simulink model "motorl"  (R2014b)
settings: Solver=ode23tb  StartTime=0.0  StopTime=1  MaxStep=.0001  MinStep=0.00001  RelTol=1e-3
libraries: powerlib x58, simulink x30, powerlib_extras x2
settings Model: Creator=Muruganandham  LastModifiedBy=SELVA
settings DataIOCC: SignalLoggingSaveFormat=ModelDataLogs
settings OptimizationCC: ExpressionDepthLimit=2147483647
settings DebuggingCC: UnderspecifiedInitializationDetection=Classic  MergeDetectMultiDrivingBlocksExec=none  FcnCallInpInsideContextMsg=UseLocalSettings  StateNameClashWarn=warning
settings GRTTargetCC: CombineOutputUpdateFcns=off  GRTInterface=on

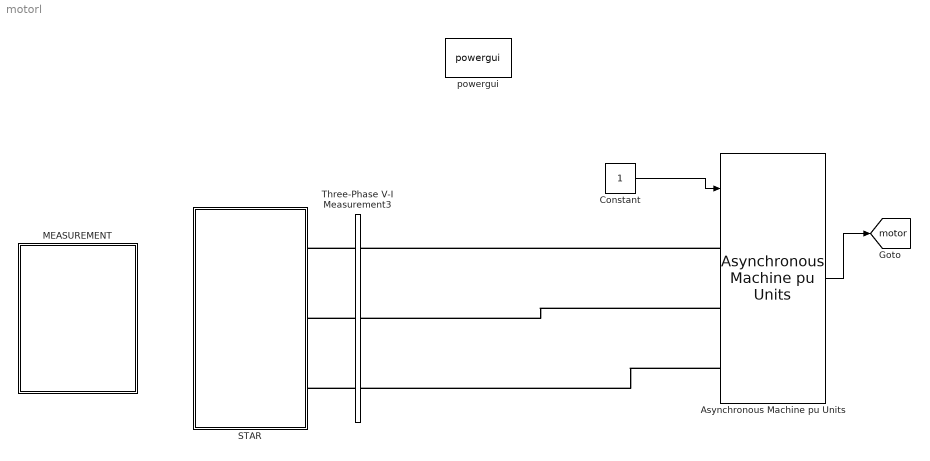
== system motorl ==
  Asynchronous Machine pu Units : powerlib/Machines/Asynchronous Machine pu Units  PresetModel="15:  5.4 HP (4KW)   400 V  50Hz 1430 RPM"  MechanicalLoad=Torque Tm  ShowDetailedParameters=on  RotorType=Squirrel-cage  ReferenceFrame=Rotor  Units=pu  MeasurementBus=off  NominalParameters=[4000 400 50]  Stator=[0.03513 0.04586]  Rotor=[0.03488 0.04586]  Cage1=[0.01909 0.0397]  Cage2=[0.01909 0.0397]  Lm=1.352  Mechanical=[0.0404 0.01841 2]  PolePairs=2  InitialConditions="[ 1,0   0,0,0   0,0,0 ]"  SimulateSaturation=off  Saturation="[0.212,0.4201,0.8125,1.0979,1.4799,2.2457,3.2586,4.5763,6.4763 ;   0.5,0.7,0.9,1,1.1,1.2 ,1.3,1.4,1.5]"  LoadFlowParameters=0  TsPowergui=0  TsBlock=-1  IterativeModel=Trapezoidal non iterative  Pmec=0
  Constant : Constant
  MEASUREMENT : Subsystem
  STAR : Subsystem  mask{v=65, fc=3000, m=1, d=0.0067}
      mask prompts: v "VOLTAGE"; fc "Switching Frequency"; m "Modulation Index"; d "Delay"
  Three-Phase V-I Measurement3 : powerlib/Measurements/Three-Phase V-I Measurement  VoltageMeasurement=phase-to-phase  SetLabelV=on  LabelV=Vabc  Vpu=off  VpuLL=off  CurrentMeasurement=yes  SetLabelI=on  LabelI=Iabc  Ipu=off  Pbase=100e6  Vbase=500e3  OutputType=Complex  PhasorSimulation=off  PSBequivalent=0
  powergui : powerlib/powergui  Priority=1  SimulationMode=Discrete  SolverType=Tustin  SampleTime=50e-6  frequency=60  SPID=off  DisableSnubberDevices=off  DisableRonSwitches=off  DisableVfSwitches=off  SwTol=0  DisplayEquations=off  Interpol=off  methode=off  Ts=0  frequencyindice=0  Pbase=100e6  ErrMax=1e-4  Iterations=50  UnitsV=kV  UnitsW=MW  FunctionMessages=off  echomessages=off  HookPort=off  EnableUseOfTLC=off  x0status=blocks  RestoreLinks=warning  ResistiveCurrentMeasurement=off  Frange=[0:2:500]  Ylog=off  Xlog=on  ShowGrid=off  save=off  variable=ZData  structure=hn  ZoomFFT=off  StartTime=0.04  cycles=7  DisplayStyle=1  fundamental=50  FreqAxis=off  MaxFrequency=1000  frequencyindicesteady=1  RmsSteady=1  display=off
  tag scope: motor=global
  wires:
  Constant/1 -> Asynchronous Machine pu Units/1
  Asynchronous Machine pu Units/1 -> [motor]
  connections:
  Asynchronous Machine pu Units/LConn3 -- Three-Phase V-I Measurement3/LConn3
  Three-Phase V-I Measurement3/RConn3 -- STAR/RConn3
  Asynchronous Machine pu Units/LConn1 -- Three-Phase V-I Measurement3/LConn1
  Three-Phase V-I Measurement3/RConn2 -- STAR/RConn2
  Three-Phase V-I Measurement3/RConn1 -- STAR/RConn1
  Asynchronous Machine pu Units/LConn2 -- Three-Phase V-I Measurement3/LConn2

== system motorl/MEASUREMENT ==
  Bus Selector : BusSelector  OutputSignals=Mechanical.Rotor speed (wm)
  Display1 : Display
  Display3 : Display
  RMS1 : powerlib_extras/Measurements/RMS  f1=50
  RMS2 : powerlib_extras/Measurements/RMS  f1=50
  Scope : Scope
      settings: YMin=-1.16  YMax=-0.96  SaveName=ScopeData5
  Scope1 : Scope
      settings: TimeRange=0.5  YMin=-800  YMax=800  SaveName=bn
  Scope2 : Scope
      settings: TimeRange=0.5  YMin=-30  YMax=30  SaveName=bn1
  wires:
  RMS2/1 -> Display3/1
  [Vabc] -> RMS2/1, Scope1/1
  [motor] -> Bus Selector/1
  Bus Selector/1 -> Scope/1  "<Rotor speed (wm)>"
  RMS1/1 -> Display1/1
  [Iabc] -> RMS1/1, Scope2/1

== system motorl/STAR ==
  "B " : Subsystem
  DC : Subsystem
  DC1 : Subsystem
  DC2 : Subsystem
  Ground : powerlib/Elements/Ground  LConnTagsString=a
  PULSE : Subsystem
  R : Subsystem
  Y : Subsystem
  A : PMIOPort  Tag=PMCPort  Port=1  Side=Right
  B : PMIOPort  Tag=PMCPort  Port=2  Side=Right
  C : PMIOPort  Tag=PMCPort  Port=3  Side=Right
  connections:
  Y/RConn2 -- Ground/LConn1 -- "B "/RConn2 -- R/RConn2
  DC/RConn1 -- R/LConn1
  DC/RConn3 -- R/LConn3
  DC/RConn4 -- R/LConn4
  DC/RConn9 -- R/LConn9
  DC/RConn2 -- R/LConn2
  DC/RConn5 -- R/LConn5
  DC/RConn7 -- R/LConn7
  DC/RConn6 -- R/LConn6
  DC/RConn8 -- R/LConn8
  DC/RConn10 -- R/LConn10
  DC1/RConn1 -- Y/LConn1
  DC1/RConn2 -- Y/LConn2
  DC1/RConn3 -- Y/LConn3
  DC1/RConn4 -- Y/LConn4
  DC1/RConn5 -- Y/LConn5
  DC1/RConn6 -- Y/LConn6
  DC1/RConn7 -- Y/LConn7
  DC1/RConn8 -- Y/LConn8
  DC1/RConn9 -- Y/LConn9
  DC1/RConn10 -- Y/LConn10
  DC2/RConn1 -- "B "/LConn1
  DC2/RConn2 -- "B "/LConn2
  DC2/RConn3 -- "B "/LConn3
  DC2/RConn4 -- "B "/LConn4
  DC2/RConn5 -- "B "/LConn5
  DC2/RConn6 -- "B "/LConn6
  DC2/RConn7 -- "B "/LConn7
  DC2/RConn8 -- "B "/LConn8
  DC2/RConn9 -- "B "/LConn9
  DC2/RConn10 -- "B "/LConn10
  A/RConn1 -- R/RConn1
  B/RConn1 -- Y/RConn1
  C/RConn1 -- "B "/RConn1

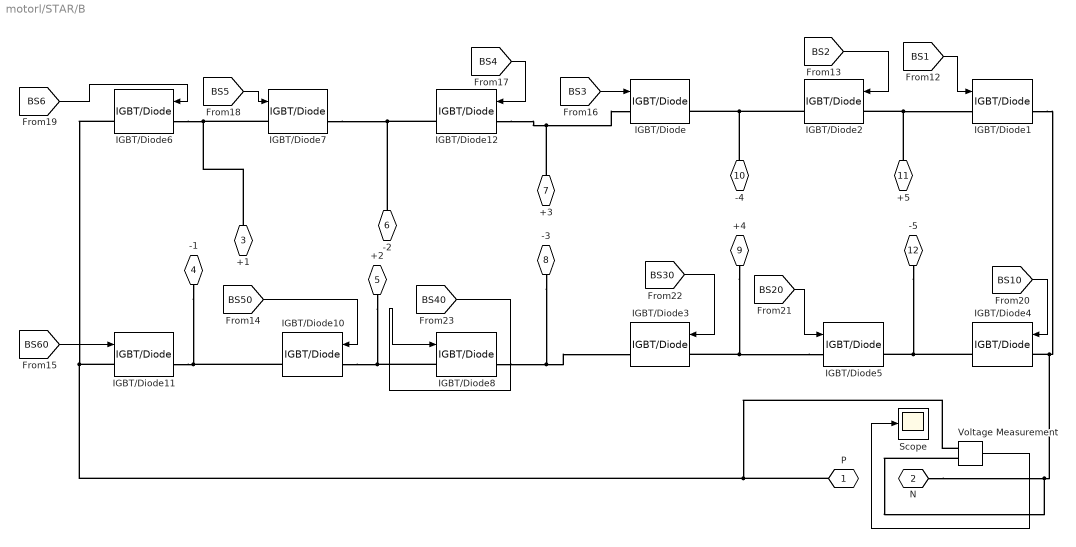
== system motorl/STAR/B  ==
  IGBT/Diode{,1..8,10..12} (12 alike) : powerlib/Power Electronics/IGBT//Diode  Ron=1e-3  Rs=1e5  Cs=inf  Measurements=on
  Scope : Scope
  Voltage Measurement : powerlib/Measurements/Voltage Measurement  PhasorSimulation=off  OutputType=Complex  PSBequivalent=0
  P : PMIOPort  Tag=PMCPort  Port=1  Side=Right
  N : PMIOPort  Tag=PMCPort  Port=2  Side=Right
  +1 : PMIOPort  Tag=PMCPort  Port=3  Side=Left
  -1 : PMIOPort  Tag=PMCPort  Port=4  Side=Left
  +2 : PMIOPort  Tag=PMCPort  Port=5  Side=Left
  -2 : PMIOPort  Tag=PMCPort  Port=6  Side=Left
  +3 : PMIOPort  Tag=PMCPort  Port=7  Side=Left
  -3 : PMIOPort  Tag=PMCPort  Port=8  Side=Left
  +4 : PMIOPort  Tag=PMCPort  Port=9  Side=Left
  -4 : PMIOPort  Tag=PMCPort  Port=10  Side=Left
  +5 : PMIOPort  Tag=PMCPort  Port=11  Side=Left
  -5 : PMIOPort  Tag=PMCPort  Port=12  Side=Left
  wires:
  [BS10] -> IGBT/Diode4/1
  [BS2] -> IGBT/Diode2/1
  [BS20] -> IGBT/Diode5/1
  [BS3] -> IGBT/Diode/1
  [BS30] -> IGBT/Diode3/1
  [BS40] -> IGBT/Diode8/1
  [BS6] -> IGBT/Diode6/1
  [BS4] -> IGBT/Diode12/1
  [BS5] -> IGBT/Diode7/1
  [BS50] -> IGBT/Diode10/1
  [BS60] -> IGBT/Diode11/1
  Voltage Measurement/1 -> Scope/1
  [BS1] -> IGBT/Diode1/1
  connections:
  IGBT/Diode2/RConn1 -- -4/RConn1 -- IGBT/Diode/RConn1
  IGBT/Diode2/LConn1 -- IGBT/Diode1/LConn1 -- +5/RConn1
  IGBT/Diode5/LConn1 -- +4/RConn1 -- IGBT/Diode3/LConn1
  IGBT/Diode4/RConn1 -- -5/RConn1 -- IGBT/Diode5/RConn1
  IGBT/Diode4/LConn1 -- IGBT/Diode1/RConn1 -- N/RConn1 -- Voltage Measurement/LConn2
  IGBT/Diode7/LConn1 -- +1/RConn1 -- IGBT/Diode6/LConn1
  IGBT/Diode12/RConn1 -- IGBT/Diode7/RConn1 -- -2/RConn1
  IGBT/Diode10/RConn1 -- IGBT/Diode11/RConn1 -- -1/RConn1
  IGBT/Diode8/LConn1 -- IGBT/Diode10/LConn1 -- +2/RConn1
  IGBT/Diode12/LConn1 -- IGBT/Diode/LConn1 -- +3/RConn1
  IGBT/Diode8/RConn1 -- IGBT/Diode3/RConn1 -- -3/RConn1
  IGBT/Diode6/RConn1 -- IGBT/Diode11/LConn1 -- P/RConn1 -- Voltage Measurement/LConn1

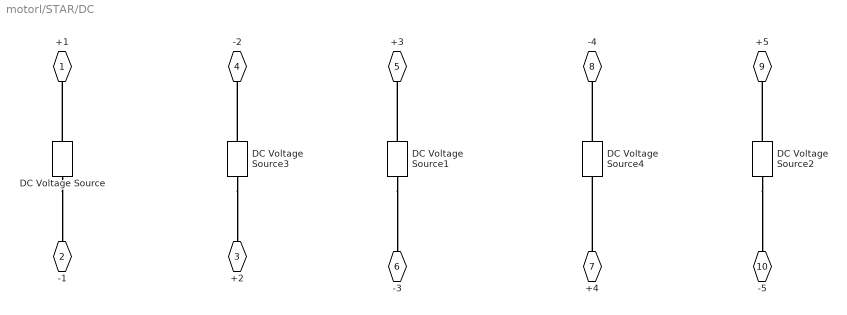
== system motorl/STAR/DC ==
  DC Voltage Source{,1..4} (5 alike) : powerlib/Electrical Sources/DC Voltage Source  Amplitude=v  Measurements=None
  +1 : PMIOPort  Tag=PMCPort  Port=1  Side=Right
  -1 : PMIOPort  Tag=PMCPort  Port=2  Side=Right
  +2 : PMIOPort  Tag=PMCPort  Port=3  Side=Right
  -2 : PMIOPort  Tag=PMCPort  Port=4  Side=Right
  +3 : PMIOPort  Tag=PMCPort  Port=5  Side=Right
  -3 : PMIOPort  Tag=PMCPort  Port=6  Side=Right
  +4 : PMIOPort  Tag=PMCPort  Port=7  Side=Right
  -4 : PMIOPort  Tag=PMCPort  Port=8  Side=Right
  +5 : PMIOPort  Tag=PMCPort  Port=9  Side=Right
  -5 : PMIOPort  Tag=PMCPort  Port=10  Side=Right
  connections:
  DC Voltage Source/LConn1 -- -1/RConn1
  DC Voltage Source/RConn1 -- +1/RConn1
  DC Voltage Source1/LConn1 -- -3/RConn1
  +4/RConn1 -- DC Voltage Source4/RConn1
  DC Voltage Source2/LConn1 -- -5/RConn1
  DC Voltage Source1/RConn1 -- +3/RConn1
  DC Voltage Source2/RConn1 -- +5/RConn1
  DC Voltage Source4/LConn1 -- -4/RConn1
  DC Voltage Source3/LConn1 -- -2/RConn1
  DC Voltage Source3/RConn1 -- +2/RConn1

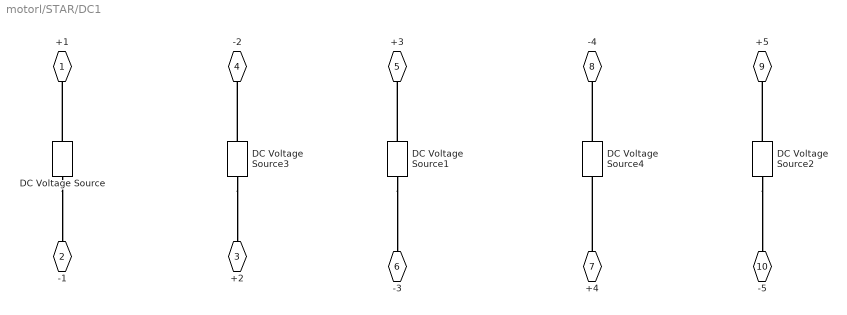
== system motorl/STAR/DC1 ==
  DC Voltage Source{,1..4} (5 alike) : powerlib/Electrical Sources/DC Voltage Source  Amplitude=v  Measurements=None
  +1 : PMIOPort  Tag=PMCPort  Port=1  Side=Right
  -1 : PMIOPort  Tag=PMCPort  Port=2  Side=Right
  +2 : PMIOPort  Tag=PMCPort  Port=3  Side=Right
  -2 : PMIOPort  Tag=PMCPort  Port=4  Side=Right
  +3 : PMIOPort  Tag=PMCPort  Port=5  Side=Right
  -3 : PMIOPort  Tag=PMCPort  Port=6  Side=Right
  +4 : PMIOPort  Tag=PMCPort  Port=7  Side=Right
  -4 : PMIOPort  Tag=PMCPort  Port=8  Side=Right
  +5 : PMIOPort  Tag=PMCPort  Port=9  Side=Right
  -5 : PMIOPort  Tag=PMCPort  Port=10  Side=Right
  connections:
  DC Voltage Source3/RConn1 -- +2/RConn1
  DC Voltage Source3/LConn1 -- -2/RConn1
  DC Voltage Source4/LConn1 -- -4/RConn1
  DC Voltage Source2/RConn1 -- +5/RConn1
  DC Voltage Source1/RConn1 -- +3/RConn1
  DC Voltage Source2/LConn1 -- -5/RConn1
  +4/RConn1 -- DC Voltage Source4/RConn1
  DC Voltage Source1/LConn1 -- -3/RConn1
  DC Voltage Source/RConn1 -- +1/RConn1
  DC Voltage Source/LConn1 -- -1/RConn1

== system motorl/STAR/DC2 ==
  DC Voltage Source{,1..4} (5 alike) : powerlib/Electrical Sources/DC Voltage Source  Amplitude=v  Measurements=None
  +1 : PMIOPort  Tag=PMCPort  Port=1  Side=Right
  -1 : PMIOPort  Tag=PMCPort  Port=2  Side=Right
  +2 : PMIOPort  Tag=PMCPort  Port=3  Side=Right
  -2 : PMIOPort  Tag=PMCPort  Port=4  Side=Right
  +3 : PMIOPort  Tag=PMCPort  Port=5  Side=Right
  -3 : PMIOPort  Tag=PMCPort  Port=6  Side=Right
  +4 : PMIOPort  Tag=PMCPort  Port=7  Side=Right
  -4 : PMIOPort  Tag=PMCPort  Port=8  Side=Right
  +5 : PMIOPort  Tag=PMCPort  Port=9  Side=Right
  -5 : PMIOPort  Tag=PMCPort  Port=10  Side=Right
  connections:
  DC Voltage Source/LConn1 -- -1/RConn1
  DC Voltage Source/RConn1 -- +1/RConn1
  DC Voltage Source1/LConn1 -- -3/RConn1
  +4/RConn1 -- DC Voltage Source4/RConn1
  DC Voltage Source2/LConn1 -- -5/RConn1
  DC Voltage Source1/RConn1 -- +3/RConn1
  DC Voltage Source2/RConn1 -- +5/RConn1
  DC Voltage Source4/LConn1 -- -4/RConn1
  DC Voltage Source3/LConn1 -- -2/RConn1
  DC Voltage Source3/RConn1 -- +2/RConn1

== system motorl/STAR/PULSE ==
  B1 : Subsystem
  R1 : Subsystem
  Y1 : Subsystem

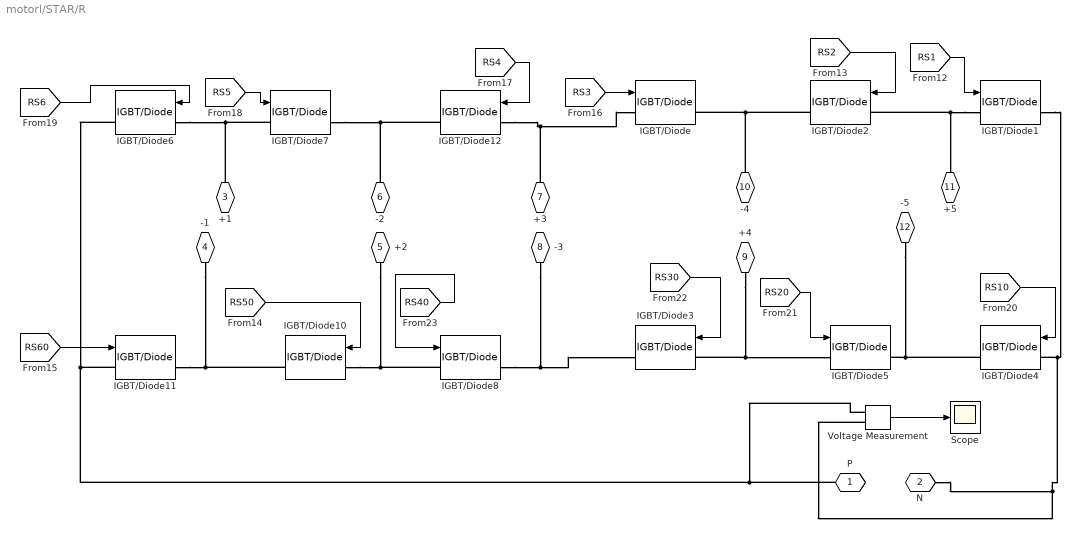
== system motorl/STAR/R ==
  IGBT/Diode{,1..8,10..12} (12 alike) : powerlib/Power Electronics/IGBT//Diode  Ron=1e-3  Rs=1e5  Cs=inf  Measurements=on
  Scope : Scope
  Voltage Measurement : powerlib/Measurements/Voltage Measurement  PhasorSimulation=off  OutputType=Complex  PSBequivalent=0
  P : PMIOPort  Tag=PMCPort  Port=1  Side=Right
  N : PMIOPort  Tag=PMCPort  Port=2  Side=Right
  +1 : PMIOPort  Tag=PMCPort  Port=3  Side=Left
  -1 : PMIOPort  Tag=PMCPort  Port=4  Side=Left
  +2 : PMIOPort  Tag=PMCPort  Port=5  Side=Left
  -2 : PMIOPort  Tag=PMCPort  Port=6  Side=Left
  +3 : PMIOPort  Tag=PMCPort  Port=7  Side=Left
  -3 : PMIOPort  Tag=PMCPort  Port=8  Side=Left
  +4 : PMIOPort  Tag=PMCPort  Port=9  Side=Left
  -4 : PMIOPort  Tag=PMCPort  Port=10  Side=Left
  +5 : PMIOPort  Tag=PMCPort  Port=11  Side=Left
  -5 : PMIOPort  Tag=PMCPort  Port=12  Side=Left
  wires:
  [RS10] -> IGBT/Diode4/1
  [RS2] -> IGBT/Diode2/1
  [RS20] -> IGBT/Diode5/1
  [RS3] -> IGBT/Diode/1
  [RS30] -> IGBT/Diode3/1
  [RS40] -> IGBT/Diode8/1
  [RS6] -> IGBT/Diode6/1
  [RS4] -> IGBT/Diode12/1
  [RS5] -> IGBT/Diode7/1
  [RS50] -> IGBT/Diode10/1
  [RS60] -> IGBT/Diode11/1
  Voltage Measurement/1 -> Scope/1
  [RS1] -> IGBT/Diode1/1
  connections:
  IGBT/Diode2/RConn1 -- -4/RConn1 -- IGBT/Diode/RConn1
  IGBT/Diode1/LConn1 -- IGBT/Diode2/LConn1 -- +5/RConn1
  +4/RConn1 -- IGBT/Diode5/LConn1 -- IGBT/Diode3/LConn1
  IGBT/Diode4/RConn1 -- -5/RConn1 -- IGBT/Diode5/RConn1
  IGBT/Diode4/LConn1 -- Voltage Measurement/LConn2 -- N/RConn1 -- IGBT/Diode1/RConn1
  IGBT/Diode7/LConn1 -- IGBT/Diode6/LConn1 -- +1/RConn1
  IGBT/Diode12/RConn1 -- -2/RConn1 -- IGBT/Diode7/RConn1
  IGBT/Diode10/RConn1 -- IGBT/Diode11/RConn1 -- -1/RConn1
  IGBT/Diode8/LConn1 -- +2/RConn1 -- IGBT/Diode10/LConn1
  IGBT/Diode12/LConn1 -- IGBT/Diode/LConn1 -- +3/RConn1
  IGBT/Diode8/RConn1 -- IGBT/Diode3/RConn1 -- -3/RConn1
  IGBT/Diode6/RConn1 -- Voltage Measurement/LConn1 -- P/RConn1 -- IGBT/Diode11/LConn1

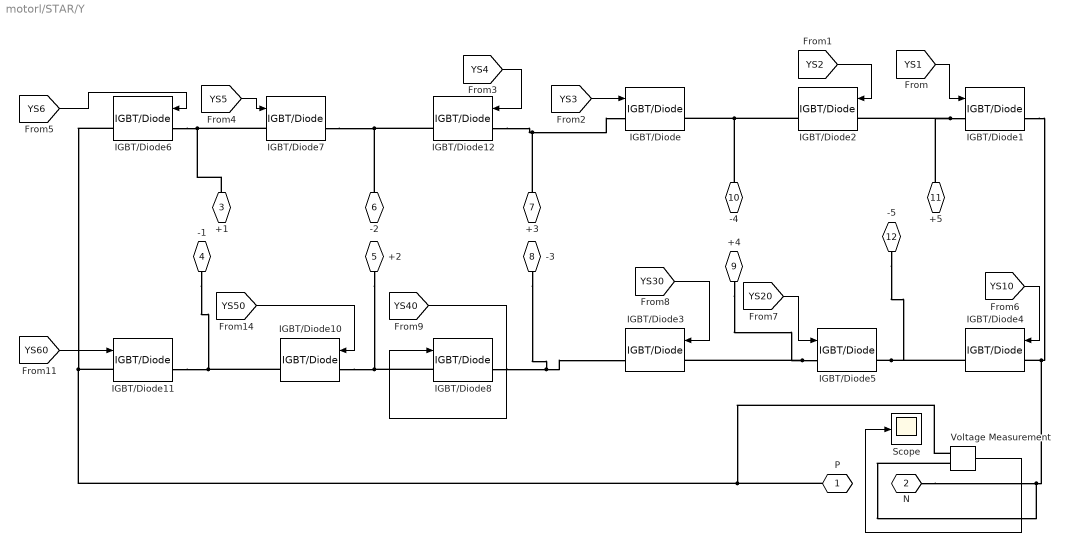
== system motorl/STAR/Y ==
  IGBT/Diode{,1..8,10..12} (12 alike) : powerlib/Power Electronics/IGBT//Diode  Ron=1e-3  Rs=1e5  Cs=inf  Measurements=on
  Scope : Scope
  Voltage Measurement : powerlib/Measurements/Voltage Measurement  PhasorSimulation=off  OutputType=Complex  PSBequivalent=0
  P : PMIOPort  Tag=PMCPort  Port=1  Side=Right
  N : PMIOPort  Tag=PMCPort  Port=2  Side=Right
  +1 : PMIOPort  Tag=PMCPort  Port=3  Side=Left
  -1 : PMIOPort  Tag=PMCPort  Port=4  Side=Left
  +2 : PMIOPort  Tag=PMCPort  Port=5  Side=Left
  -2 : PMIOPort  Tag=PMCPort  Port=6  Side=Left
  +3 : PMIOPort  Tag=PMCPort  Port=7  Side=Left
  -3 : PMIOPort  Tag=PMCPort  Port=8  Side=Left
  +4 : PMIOPort  Tag=PMCPort  Port=9  Side=Left
  -4 : PMIOPort  Tag=PMCPort  Port=10  Side=Left
  +5 : PMIOPort  Tag=PMCPort  Port=11  Side=Left
  -5 : PMIOPort  Tag=PMCPort  Port=12  Side=Left
  wires:
  [YS1] -> IGBT/Diode1/1
  Voltage Measurement/1 -> Scope/1
  [YS60] -> IGBT/Diode11/1
  [YS50] -> IGBT/Diode10/1
  [YS5] -> IGBT/Diode7/1
  [YS4] -> IGBT/Diode12/1
  [YS6] -> IGBT/Diode6/1
  [YS40] -> IGBT/Diode8/1
  [YS30] -> IGBT/Diode3/1
  [YS3] -> IGBT/Diode/1
  [YS20] -> IGBT/Diode5/1
  [YS2] -> IGBT/Diode2/1
  [YS10] -> IGBT/Diode4/1
  connections:
  Voltage Measurement/LConn1 -- P/RConn1 -- IGBT/Diode11/LConn1 -- IGBT/Diode6/RConn1
  IGBT/Diode8/RConn1 -- -3/RConn1 -- IGBT/Diode3/RConn1
  IGBT/Diode12/LConn1 -- +3/RConn1 -- IGBT/Diode/LConn1
  IGBT/Diode10/LConn1 -- IGBT/Diode8/LConn1 -- +2/RConn1
  IGBT/Diode11/RConn1 -- IGBT/Diode10/RConn1 -- -1/RConn1
  IGBT/Diode7/RConn1 -- IGBT/Diode12/RConn1 -- -2/RConn1
  IGBT/Diode6/LConn1 -- IGBT/Diode7/LConn1 -- +1/RConn1
  Voltage Measurement/LConn2 -- N/RConn1 -- IGBT/Diode1/RConn1 -- IGBT/Diode4/LConn1
  IGBT/Diode5/RConn1 -- IGBT/Diode4/RConn1 -- -5/RConn1
  IGBT/Diode5/LConn1 -- IGBT/Diode3/LConn1 -- +4/RConn1
  IGBT/Diode1/LConn1 -- IGBT/Diode2/LConn1 -- +5/RConn1
  IGBT/Diode2/RConn1 -- IGBT/Diode/RConn1 -- -4/RConn1

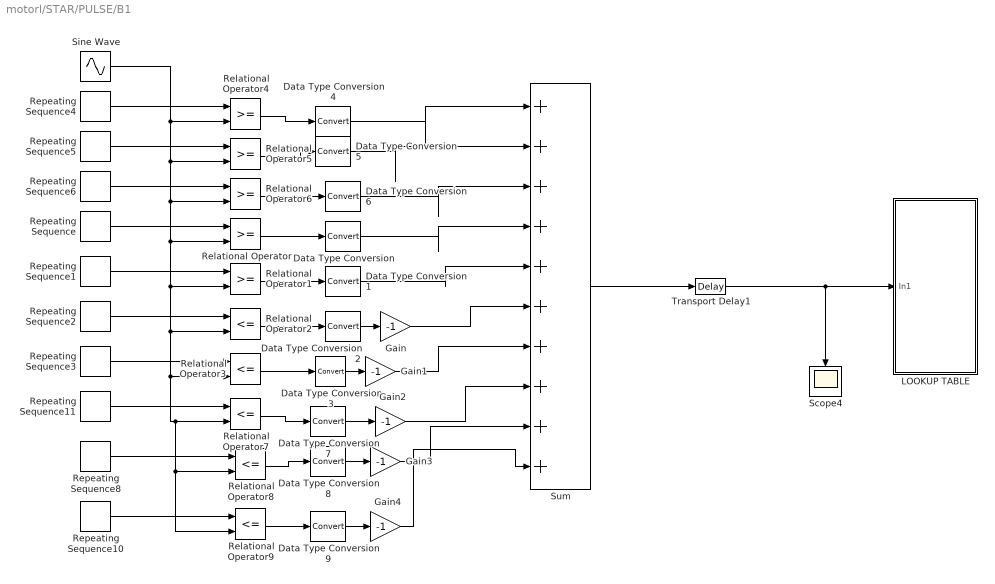
== system motorl/STAR/PULSE/B1 ==
  Data Type Conversion{,1..9} (10 alike) : DataTypeConversion
  Gain{,1..4} (5 alike) : Gain  Gain=-1
  LOOKUP TABLE : Subsystem
  Relational Operator{,1,4..6} (5 alike) : RelationalOperator  OutDataTypeStr=boolean
  Relational Operator{2..3,7..9} (5 alike) : RelationalOperator  Operator=<=  OutDataTypeStr=boolean
  Repeating Sequence : simulink/Sources/Repeating Sequence  rep_seq_t="[0 (1/fc)/2  (1/fc)]"  rep_seq_y=[2 1 2]
  Repeating Sequence1 : simulink/Sources/Repeating Sequence  rep_seq_t="[0 (1/fc)/2  (1/fc)]"  rep_seq_y=[1 0 1]
  Repeating Sequence10 : simulink/Sources/Repeating Sequence  rep_seq_t="[0 (0.1/fc)/2  (0.1/fc)]"  rep_seq_y=[-5 -4 -5]
  Repeating Sequence11 : simulink/Sources/Repeating Sequence  rep_seq_t="[0 (1/fc)/2  (1/fc)]"  rep_seq_y=[-3 -2 -3]
  Repeating Sequence2 : simulink/Sources/Repeating Sequence  rep_seq_t="[0 (1/fc)/2  (1/fc)]"  rep_seq_y=[-1 0 -1]
  Repeating Sequence3 : simulink/Sources/Repeating Sequence  rep_seq_t="[0 (1/fc)/2  (1/fc)]"  rep_seq_y=[-2 -1 -2]
  Repeating Sequence4 : simulink/Sources/Repeating Sequence  rep_seq_t="[0 (0.1/fc)/2  (0.1/fc)]"  rep_seq_y=[4 5 4]
  Repeating Sequence5 : simulink/Sources/Repeating Sequence  rep_seq_t="[0 (1/fc)/2  (1/fc)]"  rep_seq_y=[4 3 4]
  Repeating Sequence6 : simulink/Sources/Repeating Sequence  rep_seq_t="[0 (1/fc)/2  (1/fc)]"  rep_seq_y=[3 2 3]
  Repeating Sequence8 : simulink/Sources/Repeating Sequence  rep_seq_t="[0 (1/fc)/2  (1/fc)]"  rep_seq_y=[-4 -3 -4]
  Scope4 : Scope
      settings: SaveName=ScopeData8
  Sine Wave : Sin  Amplitude=5*m  Frequency=2*pi*50  SampleTime=0
  Sum : Sum  Inputs=|++++++++++
  Transport Delay1 : TransportDelay  DelayTime=2*d
  wires:
  Data Type Conversion3/1 -> Gain1/1
  Data Type Conversion2/1 -> Gain/1
  Relational Operator3/1 -> Data Type Conversion3/1
  Relational Operator2/1 -> Data Type Conversion2/1
  Repeating Sequence3/1 -> Relational Operator3/1
  Repeating Sequence2/1 -> Relational Operator2/1
  Repeating Sequence1/1 -> Relational Operator1/1
  Repeating Sequence/1 -> Relational Operator/1
  Relational Operator1/1 -> Data Type Conversion1/1
  Relational Operator/1 -> Data Type Conversion/1
  Repeating Sequence6/1 -> Relational Operator6/1
  Repeating Sequence5/1 -> Relational Operator5/1
  Repeating Sequence4/1 -> Relational Operator4/1
  Relational Operator6/1 -> Data Type Conversion6/1
  Relational Operator5/1 -> Data Type Conversion5/1
  Relational Operator4/1 -> Data Type Conversion4/1
  Repeating Sequence8/1 -> Relational Operator8/1
  Repeating Sequence11/1 -> Relational Operator7/1
  Relational Operator9/1 -> Data Type Conversion9/1
  Relational Operator8/1 -> Data Type Conversion8/1
  Relational Operator7/1 -> Data Type Conversion7/1
  Data Type Conversion9/1 -> Gain4/1
  Data Type Conversion8/1 -> Gain3/1
  Data Type Conversion7/1 -> Gain2/1
  Repeating Sequence10/1 -> Relational Operator9/1
  Data Type Conversion4/1 -> Sum/1
  Data Type Conversion5/1 -> Sum/2
  Data Type Conversion6/1 -> Sum/3
  Data Type Conversion/1 -> Sum/4
  Data Type Conversion1/1 -> Sum/5
  Gain/1 -> Sum/6
  Gain1/1 -> Sum/7
  Gain2/1 -> Sum/8
  Gain3/1 -> Sum/9
  Gain4/1 -> Sum/10
  Sine Wave/1 -> Relational Operator5/2, Relational Operator6/2, Relational Operator/2, Relational Operator1/2, Relational Operator2/2, Relational Operator3/2, Relational Operator7/2, Relational Operator9/2, Relational Operator8/2, Relational Operator4/2
  Sum/1 -> Transport Delay1/1
  Transport Delay1/1 -> Scope4/1, LOOKUP TABLE/1(In1)

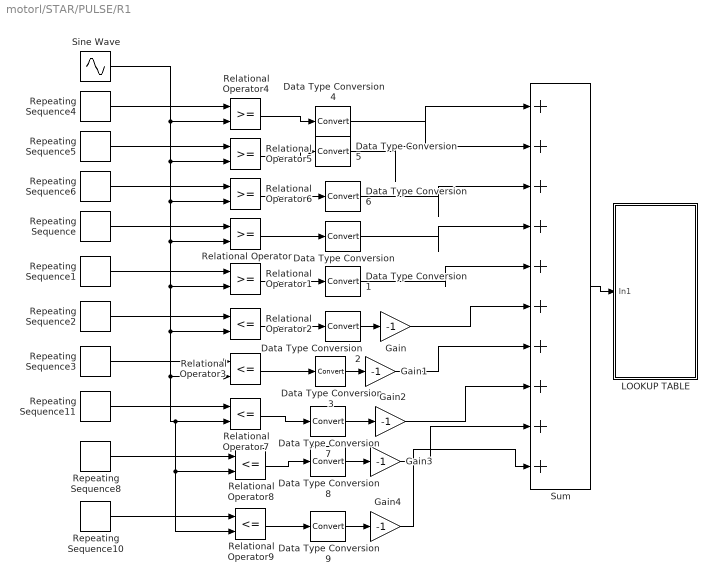
== system motorl/STAR/PULSE/R1 ==
  Data Type Conversion{,1..9} (10 alike) : DataTypeConversion
  Gain{,1..4} (5 alike) : Gain  Gain=-1
  LOOKUP TABLE : Subsystem
  Relational Operator{,1,4..6} (5 alike) : RelationalOperator  OutDataTypeStr=boolean
  Relational Operator{2..3,7..9} (5 alike) : RelationalOperator  Operator=<=  OutDataTypeStr=boolean
  Repeating Sequence : simulink/Sources/Repeating Sequence  rep_seq_t="[0 (1/fc)/2  (1/fc)]"  rep_seq_y=[2 1 2]
  Repeating Sequence1 : simulink/Sources/Repeating Sequence  rep_seq_t="[0 (1/fc)/2  (1/fc)]"  rep_seq_y=[1 0 1]
  Repeating Sequence10 : simulink/Sources/Repeating Sequence  rep_seq_t="[0 (0.1/fc)/2  (0.1/fc)]"  rep_seq_y=[-5 -4 -5]
  Repeating Sequence11 : simulink/Sources/Repeating Sequence  rep_seq_t="[0 (1/fc)/2  (1/fc)]"  rep_seq_y=[-3 -2 -3]
  Repeating Sequence2 : simulink/Sources/Repeating Sequence  rep_seq_t="[0 (1/fc)/2  (1/fc)]"  rep_seq_y=[-1 0 -1]
  Repeating Sequence3 : simulink/Sources/Repeating Sequence  rep_seq_t="[0 (1/fc)/2  (1/fc)]"  rep_seq_y=[-2 -1 -2]
  Repeating Sequence4 : simulink/Sources/Repeating Sequence  rep_seq_t="[0 (0.1/fc)/2  (0.1/fc)]"  rep_seq_y=[4 5 4]
  Repeating Sequence5 : simulink/Sources/Repeating Sequence  rep_seq_t="[0 (1/fc)/2  (1/fc)]"  rep_seq_y=[4 3 4]
  Repeating Sequence6 : simulink/Sources/Repeating Sequence  rep_seq_t="[0 (1/fc)/2  (1/fc)]"  rep_seq_y=[3 2 3]
  Repeating Sequence8 : simulink/Sources/Repeating Sequence  rep_seq_t="[0 (1/fc)/2  (1/fc)]"  rep_seq_y=[-4 -3 -4]
  Sine Wave : Sin  Amplitude=5*m  Frequency=2*pi*50  SampleTime=0
  Sum : Sum  Inputs=|++++++++++
  wires:
  Data Type Conversion3/1 -> Gain1/1
  Data Type Conversion2/1 -> Gain/1
  Relational Operator3/1 -> Data Type Conversion3/1
  Relational Operator2/1 -> Data Type Conversion2/1
  Repeating Sequence3/1 -> Relational Operator3/1
  Repeating Sequence2/1 -> Relational Operator2/1
  Repeating Sequence1/1 -> Relational Operator1/1
  Repeating Sequence/1 -> Relational Operator/1
  Relational Operator1/1 -> Data Type Conversion1/1
  Relational Operator/1 -> Data Type Conversion/1
  Repeating Sequence6/1 -> Relational Operator6/1
  Repeating Sequence5/1 -> Relational Operator5/1
  Repeating Sequence4/1 -> Relational Operator4/1
  Relational Operator6/1 -> Data Type Conversion6/1
  Relational Operator5/1 -> Data Type Conversion5/1
  Relational Operator4/1 -> Data Type Conversion4/1
  Repeating Sequence8/1 -> Relational Operator8/1
  Repeating Sequence11/1 -> Relational Operator7/1
  Relational Operator9/1 -> Data Type Conversion9/1
  Relational Operator8/1 -> Data Type Conversion8/1
  Relational Operator7/1 -> Data Type Conversion7/1
  Data Type Conversion9/1 -> Gain4/1
  Data Type Conversion8/1 -> Gain3/1
  Data Type Conversion7/1 -> Gain2/1
  Repeating Sequence10/1 -> Relational Operator9/1
  Data Type Conversion4/1 -> Sum/1
  Data Type Conversion5/1 -> Sum/2
  Data Type Conversion6/1 -> Sum/3
  Data Type Conversion/1 -> Sum/4
  Data Type Conversion1/1 -> Sum/5
  Gain/1 -> Sum/6
  Gain1/1 -> Sum/7
  Gain2/1 -> Sum/8
  Gain3/1 -> Sum/9
  Gain4/1 -> Sum/10
  Sum/1 -> LOOKUP TABLE/1(In1)
  Sine Wave/1 -> Relational Operator5/2, Relational Operator6/2, Relational Operator/2, Relational Operator1/2, Relational Operator2/2, Relational Operator3/2, Relational Operator7/2, Relational Operator9/2, Relational Operator8/2, Relational Operator4/2

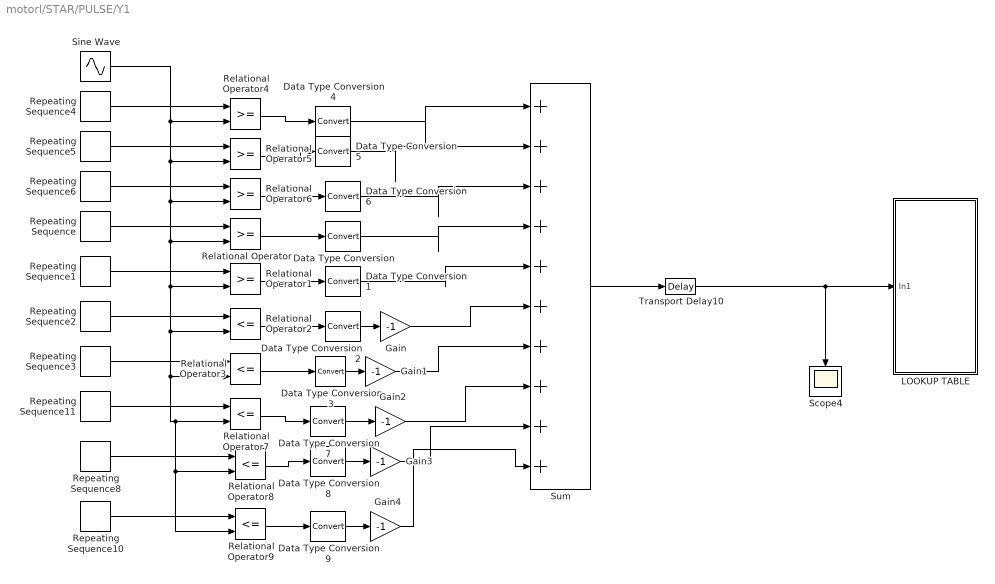
== system motorl/STAR/PULSE/Y1 ==
  Data Type Conversion{,1..9} (10 alike) : DataTypeConversion
  Gain{,1..4} (5 alike) : Gain  Gain=-1
  LOOKUP TABLE : Subsystem
  Relational Operator{,1,4..6} (5 alike) : RelationalOperator  OutDataTypeStr=boolean
  Relational Operator{2..3,7..9} (5 alike) : RelationalOperator  Operator=<=  OutDataTypeStr=boolean
  Repeating Sequence : simulink/Sources/Repeating Sequence  rep_seq_t="[0 (1/fc)/2  (1/fc)]"  rep_seq_y=[2 1 2]
  Repeating Sequence1 : simulink/Sources/Repeating Sequence  rep_seq_t="[0 (1/fc)/2  (1/fc)]"  rep_seq_y=[1 0 1]
  Repeating Sequence10 : simulink/Sources/Repeating Sequence  rep_seq_t="[0 (0.1/fc)/2  (0.1/fc)]"  rep_seq_y=[-5 -4 -5]
  Repeating Sequence11 : simulink/Sources/Repeating Sequence  rep_seq_t="[0 (1/fc)/2  (1/fc)]"  rep_seq_y=[-3 -2 -3]
  Repeating Sequence2 : simulink/Sources/Repeating Sequence  rep_seq_t="[0 (1/fc)/2  (1/fc)]"  rep_seq_y=[-1 0 -1]
  Repeating Sequence3 : simulink/Sources/Repeating Sequence  rep_seq_t="[0 (1/fc)/2  (1/fc)]"  rep_seq_y=[-2 -1 -2]
  Repeating Sequence4 : simulink/Sources/Repeating Sequence  rep_seq_t="[0 (0.1/fc)/2  (0.1/fc)]"  rep_seq_y=[4 5 4]
  Repeating Sequence5 : simulink/Sources/Repeating Sequence  rep_seq_t="[0 (1/fc)/2  (1/fc)]"  rep_seq_y=[4 3 4]
  Repeating Sequence6 : simulink/Sources/Repeating Sequence  rep_seq_t="[0 (1/fc)/2  (1/fc)]"  rep_seq_y=[3 2 3]
  Repeating Sequence8 : simulink/Sources/Repeating Sequence  rep_seq_t="[0 (1/fc)/2  (1/fc)]"  rep_seq_y=[-4 -3 -4]
  Scope4 : Scope
      settings: SaveName=ScopeData8
  Sine Wave : Sin  Amplitude=5*m  Frequency=2*pi*50  SampleTime=0
  Sum : Sum  Inputs=|++++++++++
  Transport Delay10 : TransportDelay  DelayTime=d
  wires:
  Sum/1 -> Transport Delay10/1
  Sine Wave/1 -> Relational Operator4/2, Relational Operator8/2, Relational Operator9/2, Relational Operator7/2, Relational Operator3/2, Relational Operator2/2, Relational Operator1/2, Relational Operator/2, Relational Operator6/2, Relational Operator5/2
  Gain4/1 -> Sum/10
  Gain3/1 -> Sum/9
  Gain2/1 -> Sum/8
  Gain1/1 -> Sum/7
  Gain/1 -> Sum/6
  Data Type Conversion1/1 -> Sum/5
  Data Type Conversion/1 -> Sum/4
  Data Type Conversion6/1 -> Sum/3
  Data Type Conversion5/1 -> Sum/2
  Data Type Conversion4/1 -> Sum/1
  Data Type Conversion7/1 -> Gain2/1
  Data Type Conversion8/1 -> Gain3/1
  Data Type Conversion9/1 -> Gain4/1
  Relational Operator7/1 -> Data Type Conversion7/1
  Relational Operator8/1 -> Data Type Conversion8/1
  Relational Operator9/1 -> Data Type Conversion9/1
  Relational Operator4/1 -> Data Type Conversion4/1
  Relational Operator5/1 -> Data Type Conversion5/1
  Relational Operator6/1 -> Data Type Conversion6/1
  Relational Operator/1 -> Data Type Conversion/1
  Relational Operator1/1 -> Data Type Conversion1/1
  Relational Operator2/1 -> Data Type Conversion2/1
  Relational Operator3/1 -> Data Type Conversion3/1
  Data Type Conversion2/1 -> Gain/1
  Data Type Conversion3/1 -> Gain1/1
  Repeating Sequence4/1 -> Relational Operator4/1
  Repeating Sequence5/1 -> Relational Operator5/1
  Repeating Sequence6/1 -> Relational Operator6/1
  Repeating Sequence/1 -> Relational Operator/1
  Repeating Sequence1/1 -> Relational Operator1/1
  Repeating Sequence2/1 -> Relational Operator2/1
  Repeating Sequence3/1 -> Relational Operator3/1
  Repeating Sequence11/1 -> Relational Operator7/1
  Repeating Sequence8/1 -> Relational Operator8/1
  Repeating Sequence10/1 -> Relational Operator9/1
  Transport Delay10/1 -> LOOKUP TABLE/1(In1), Scope4/1

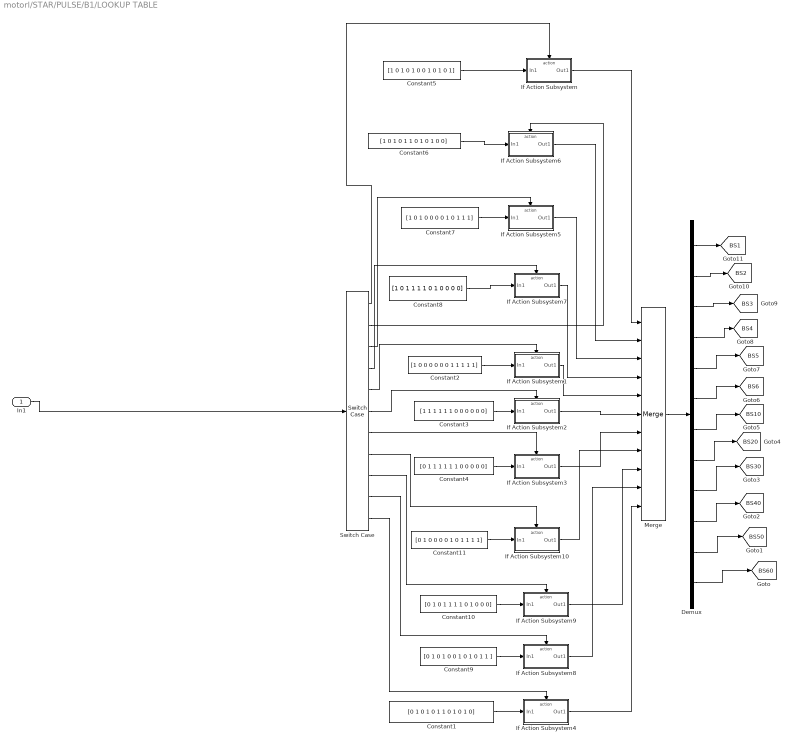
== system motorl/STAR/PULSE/B1/LOOKUP TABLE ==
  In1 : Inport
  Constant1 : Constant  Value=[0 1 0 1 0 1 1 0 1 0 1 0]
  Constant10 : Constant  Value=[0 1 0 1 1 1 1 0 1 0 0 0]
  Constant11 : Constant  Value=[0 1 0 0 0 0 1 0 1 1 1 1]
  Constant2 : Constant  Value=[1 0 0 0 0 0 0 1 1 1 1 1]
  Constant3 : Constant  Value=[1 1 1 1 1 1 0 0 0 0 0 0]
  Constant4 : Constant  Value=[0 1 1 1 1 1 1 0 0 0 0 0]
  Constant5 : Constant  Value=[1 0 1 0 1 0 0 1 0 1 0 1]
  Constant6 : Constant  Value=[1 0 1 0 1 1 0 1 0 1 0 0]
  Constant7 : Constant  Value=[1 0 1 0 0 0 0 1 0 1 1 1]
  Constant8 : Constant  Value=[1 0 1 1 1 1 0 1 0 0 0 0]
  Constant9 : Constant  Value=[0 1 0 1 0 0 1 0 1 0 1 1 ]
  Demux : Demux  Outputs=12
  If Action Subsystem : Subsystem  TreatAsAtomicUnit=on
  If Action Subsystem1 : Subsystem  TreatAsAtomicUnit=on
  If Action Subsystem10 : Subsystem  TreatAsAtomicUnit=on
  If Action Subsystem2 : Subsystem  TreatAsAtomicUnit=on
  If Action Subsystem3 : Subsystem  TreatAsAtomicUnit=on
  If Action Subsystem4 : Subsystem  TreatAsAtomicUnit=on
  If Action Subsystem5 : Subsystem  TreatAsAtomicUnit=on
  If Action Subsystem6 : Subsystem  TreatAsAtomicUnit=on
  If Action Subsystem7 : Subsystem  TreatAsAtomicUnit=on
  If Action Subsystem8 : Subsystem  TreatAsAtomicUnit=on
  If Action Subsystem9 : Subsystem  TreatAsAtomicUnit=on
  Merge : Merge  Inputs=11
  Switch Case : SwitchCase  CaseConditions={-5 -4 -3 -2 -1 0 1 2 3 4 5}  ShowDefaultCase=off
  tag scope: BS10=global, BS1=global, BS20=global, BS2=global, BS30=global, BS3=global, BS40=global, BS4=global, BS50=global, BS5=global, BS60=global, BS6=global
  wires:
  Merge/1 -> Demux/1
  If Action Subsystem/1(Out1) -> Merge/1
  Constant4/1 -> If Action Subsystem3/1(In1)
  Constant3/1 -> If Action Subsystem2/1(In1)
  Constant2/1 -> If Action Subsystem1/1(In1)
  Switch Case/6 -> If Action Subsystem2/Action
  If Action Subsystem6/1(Out1) -> Merge/2
  If Action Subsystem5/1(Out1) -> Merge/3
  If Action Subsystem7/1(Out1) -> Merge/4
  If Action Subsystem1/1(Out1) -> Merge/5
  If Action Subsystem2/1(Out1) -> Merge/6
  If Action Subsystem3/1(Out1) -> Merge/7
  Constant9/1 -> If Action Subsystem8/1(In1)
  Constant10/1 -> If Action Subsystem9/1(In1)
  Constant11/1 -> If Action Subsystem10/1(In1)
  Switch Case/11 -> If Action Subsystem4/Action
  If Action Subsystem4/1(Out1) -> Merge/11
  Switch Case/10 -> If Action Subsystem8/Action
  Switch Case/9 -> If Action Subsystem9/Action
  Switch Case/8 -> If Action Subsystem10/Action
  Switch Case/7 -> If Action Subsystem3/Action
  Switch Case/5 -> If Action Subsystem1/Action
  Switch Case/4 -> If Action Subsystem7/Action
  Switch Case/3 -> If Action Subsystem5/Action
  Switch Case/2 -> If Action Subsystem6/Action
  Switch Case/1 -> If Action Subsystem/Action
  Constant6/1 -> If Action Subsystem6/1(In1)
  Constant7/1 -> If Action Subsystem5/1(In1)
  Constant8/1 -> If Action Subsystem7/1(In1)
  If Action Subsystem10/1(Out1) -> Merge/8
  If Action Subsystem9/1(Out1) -> Merge/9
  If Action Subsystem8/1(Out1) -> Merge/10
  Constant1/1 -> If Action Subsystem4/1(In1)
  Constant5/1 -> If Action Subsystem/1(In1)
  In1/1 -> Switch Case/1
  Demux/1 -> [BS1]
  Demux/2 -> [BS2]
  Demux/3 -> [BS3]
  Demux/4 -> [BS4]
  Demux/6 -> [BS6]
  Demux/5 -> [BS5]
  Demux/7 -> [BS10]
  Demux/8 -> [BS20]
  Demux/11 -> [BS50]
  Demux/10 -> [BS40]
  Demux/9 -> [BS30]
  Demux/12 -> [BS60]

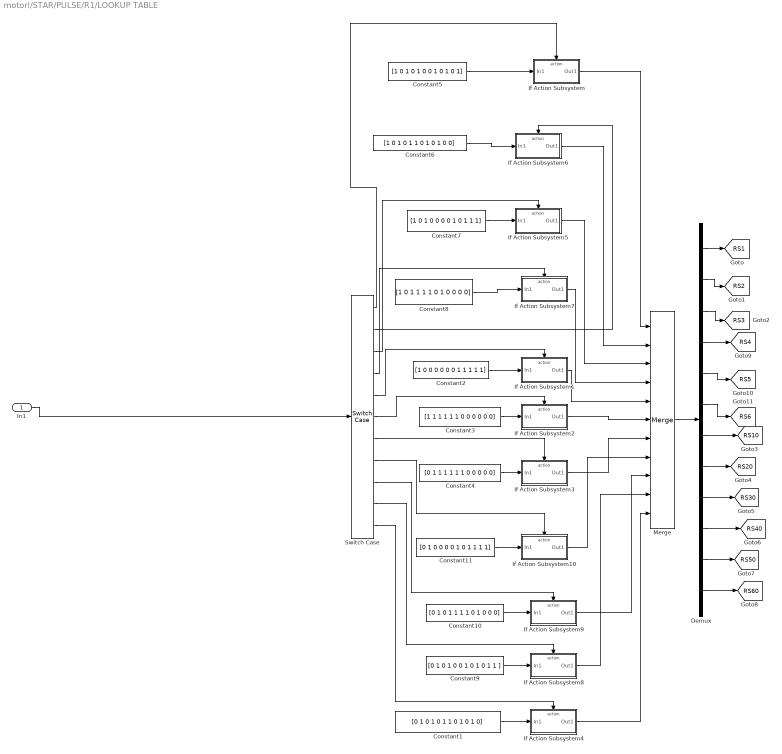
== system motorl/STAR/PULSE/R1/LOOKUP TABLE ==
  In1 : Inport
  Constant1 : Constant  Value=[0 1 0 1 0 1 1 0 1 0 1 0]
  Constant10 : Constant  Value=[0 1 0 1 1 1 1 0 1 0 0 0]
  Constant11 : Constant  Value=[0 1 0 0 0 0 1 0 1 1 1 1]
  Constant2 : Constant  Value=[1 0 0 0 0 0 0 1 1 1 1 1]
  Constant3 : Constant  Value=[1 1 1 1 1 1 0 0 0 0 0 0]
  Constant4 : Constant  Value=[0 1 1 1 1 1 1 0 0 0 0 0]
  Constant5 : Constant  Value=[1 0 1 0 1 0 0 1 0 1 0 1]
  Constant6 : Constant  Value=[1 0 1 0 1 1 0 1 0 1 0 0]
  Constant7 : Constant  Value=[1 0 1 0 0 0 0 1 0 1 1 1]
  Constant8 : Constant  Value=[1 0 1 1 1 1 0 1 0 0 0 0]
  Constant9 : Constant  Value=[0 1 0 1 0 0 1 0 1 0 1 1 ]
  Demux : Demux  Outputs=12
  If Action Subsystem : Subsystem  TreatAsAtomicUnit=on
  If Action Subsystem1 : Subsystem  TreatAsAtomicUnit=on
  If Action Subsystem10 : Subsystem  TreatAsAtomicUnit=on
  If Action Subsystem2 : Subsystem  TreatAsAtomicUnit=on
  If Action Subsystem3 : Subsystem  TreatAsAtomicUnit=on
  If Action Subsystem4 : Subsystem  TreatAsAtomicUnit=on
  If Action Subsystem5 : Subsystem  TreatAsAtomicUnit=on
  If Action Subsystem6 : Subsystem  TreatAsAtomicUnit=on
  If Action Subsystem7 : Subsystem  TreatAsAtomicUnit=on
  If Action Subsystem8 : Subsystem  TreatAsAtomicUnit=on
  If Action Subsystem9 : Subsystem  TreatAsAtomicUnit=on
  Merge : Merge  Inputs=11
  Switch Case : SwitchCase  CaseConditions={-5 -4 -3 -2 -1 0 1 2 3 4 5}  ShowDefaultCase=off
  tag scope: RS10=global, RS1=global, RS20=global, RS2=global, RS30=global, RS3=global, RS40=global, RS4=global, RS50=global, RS5=global, RS60=global, RS6=global
  wires:
  Merge/1 -> Demux/1
  If Action Subsystem/1(Out1) -> Merge/1
  Constant4/1 -> If Action Subsystem3/1(In1)
  Constant3/1 -> If Action Subsystem2/1(In1)
  Constant2/1 -> If Action Subsystem1/1(In1)
  Switch Case/6 -> If Action Subsystem2/Action
  If Action Subsystem6/1(Out1) -> Merge/2
  If Action Subsystem5/1(Out1) -> Merge/3
  If Action Subsystem7/1(Out1) -> Merge/4
  If Action Subsystem1/1(Out1) -> Merge/5
  If Action Subsystem2/1(Out1) -> Merge/6
  If Action Subsystem3/1(Out1) -> Merge/7
  Constant9/1 -> If Action Subsystem8/1(In1)
  Constant10/1 -> If Action Subsystem9/1(In1)
  Constant11/1 -> If Action Subsystem10/1(In1)
  Switch Case/11 -> If Action Subsystem4/Action
  If Action Subsystem4/1(Out1) -> Merge/11
  Switch Case/10 -> If Action Subsystem8/Action
  Switch Case/9 -> If Action Subsystem9/Action
  Switch Case/8 -> If Action Subsystem10/Action
  Switch Case/7 -> If Action Subsystem3/Action
  Switch Case/5 -> If Action Subsystem1/Action
  Switch Case/4 -> If Action Subsystem7/Action
  Switch Case/3 -> If Action Subsystem5/Action
  Switch Case/2 -> If Action Subsystem6/Action
  Switch Case/1 -> If Action Subsystem/Action
  Constant6/1 -> If Action Subsystem6/1(In1)
  Constant7/1 -> If Action Subsystem5/1(In1)
  Constant8/1 -> If Action Subsystem7/1(In1)
  If Action Subsystem10/1(Out1) -> Merge/8
  If Action Subsystem9/1(Out1) -> Merge/9
  If Action Subsystem8/1(Out1) -> Merge/10
  Demux/3 -> [RS3]
  Demux/2 -> [RS2]
  Demux/1 -> [RS1]
  Demux/7 -> [RS10]
  Demux/8 -> [RS20]
  Demux/9 -> [RS30]
  Demux/10 -> [RS40]
  Demux/11 -> [RS50]
  Demux/12 -> [RS60]
  Demux/6 -> [RS6]
  Demux/5 -> [RS5]
  Demux/4 -> [RS4]
  Constant1/1 -> If Action Subsystem4/1(In1)
  Constant5/1 -> If Action Subsystem/1(In1)
  In1/1 -> Switch Case/1

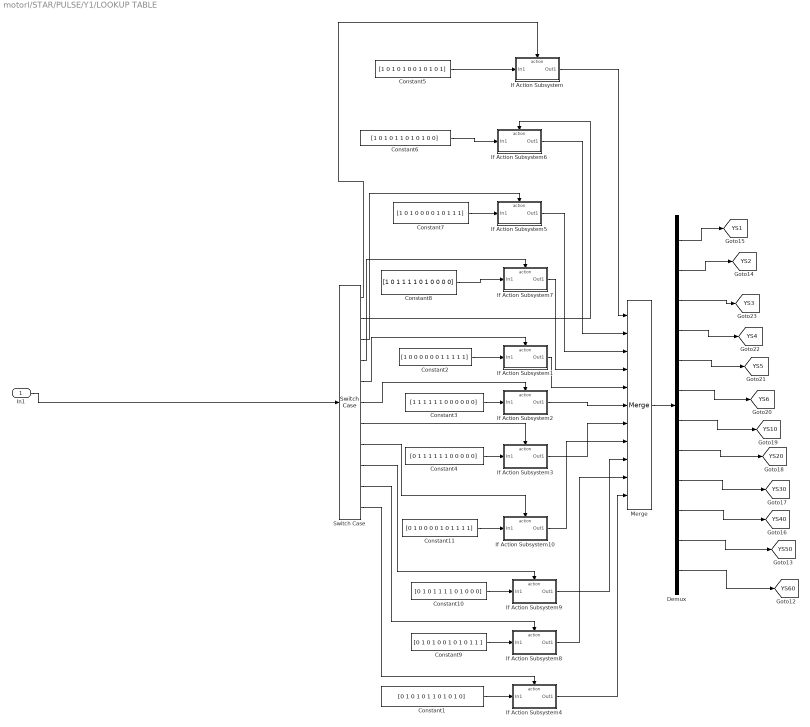
== system motorl/STAR/PULSE/Y1/LOOKUP TABLE ==
  In1 : Inport
  Constant1 : Constant  Value=[0 1 0 1 0 1 1 0 1 0 1 0]
  Constant10 : Constant  Value=[0 1 0 1 1 1 1 0 1 0 0 0]
  Constant11 : Constant  Value=[0 1 0 0 0 0 1 0 1 1 1 1]
  Constant2 : Constant  Value=[1 0 0 0 0 0 0 1 1 1 1 1]
  Constant3 : Constant  Value=[1 1 1 1 1 1 0 0 0 0 0 0]
  Constant4 : Constant  Value=[0 1 1 1 1 1 1 0 0 0 0 0]
  Constant5 : Constant  Value=[1 0 1 0 1 0 0 1 0 1 0 1]
  Constant6 : Constant  Value=[1 0 1 0 1 1 0 1 0 1 0 0]
  Constant7 : Constant  Value=[1 0 1 0 0 0 0 1 0 1 1 1]
  Constant8 : Constant  Value=[1 0 1 1 1 1 0 1 0 0 0 0]
  Constant9 : Constant  Value=[0 1 0 1 0 0 1 0 1 0 1 1 ]
  Demux : Demux  Outputs=12
  If Action Subsystem : Subsystem  TreatAsAtomicUnit=on
  If Action Subsystem1 : Subsystem  TreatAsAtomicUnit=on
  If Action Subsystem10 : Subsystem  TreatAsAtomicUnit=on
  If Action Subsystem2 : Subsystem  TreatAsAtomicUnit=on
  If Action Subsystem3 : Subsystem  TreatAsAtomicUnit=on
  If Action Subsystem4 : Subsystem  TreatAsAtomicUnit=on
  If Action Subsystem5 : Subsystem  TreatAsAtomicUnit=on
  If Action Subsystem6 : Subsystem  TreatAsAtomicUnit=on
  If Action Subsystem7 : Subsystem  TreatAsAtomicUnit=on
  If Action Subsystem8 : Subsystem  TreatAsAtomicUnit=on
  If Action Subsystem9 : Subsystem  TreatAsAtomicUnit=on
  Merge : Merge  Inputs=11
  Switch Case : SwitchCase  CaseConditions={-5 -4 -3 -2 -1 0 1 2 3 4 5}  ShowDefaultCase=off
  tag scope: YS10=global, YS1=global, YS20=global, YS2=global, YS30=global, YS3=global, YS40=global, YS4=global, YS50=global, YS5=global, YS60=global, YS6=global
  wires:
  In1/1 -> Switch Case/1
  Constant5/1 -> If Action Subsystem/1(In1)
  Constant1/1 -> If Action Subsystem4/1(In1)
  If Action Subsystem8/1(Out1) -> Merge/10
  If Action Subsystem9/1(Out1) -> Merge/9
  If Action Subsystem10/1(Out1) -> Merge/8
  Constant8/1 -> If Action Subsystem7/1(In1)
  Constant7/1 -> If Action Subsystem5/1(In1)
  Constant6/1 -> If Action Subsystem6/1(In1)
  Switch Case/1 -> If Action Subsystem/Action
  Switch Case/2 -> If Action Subsystem6/Action
  Switch Case/3 -> If Action Subsystem5/Action
  Switch Case/4 -> If Action Subsystem7/Action
  Switch Case/5 -> If Action Subsystem1/Action
  Switch Case/7 -> If Action Subsystem3/Action
  Switch Case/8 -> If Action Subsystem10/Action
  Switch Case/9 -> If Action Subsystem9/Action
  Switch Case/10 -> If Action Subsystem8/Action
  If Action Subsystem4/1(Out1) -> Merge/11
  Switch Case/11 -> If Action Subsystem4/Action
  Constant11/1 -> If Action Subsystem10/1(In1)
  Constant10/1 -> If Action Subsystem9/1(In1)
  Constant9/1 -> If Action Subsystem8/1(In1)
  If Action Subsystem3/1(Out1) -> Merge/7
  If Action Subsystem2/1(Out1) -> Merge/6
  If Action Subsystem1/1(Out1) -> Merge/5
  If Action Subsystem7/1(Out1) -> Merge/4
  If Action Subsystem5/1(Out1) -> Merge/3
  If Action Subsystem6/1(Out1) -> Merge/2
  Switch Case/6 -> If Action Subsystem2/Action
  Constant2/1 -> If Action Subsystem1/1(In1)
  Constant3/1 -> If Action Subsystem2/1(In1)
  Constant4/1 -> If Action Subsystem3/1(In1)
  If Action Subsystem/1(Out1) -> Merge/1
  Merge/1 -> Demux/1
  Demux/1 -> [YS1]
  Demux/3 -> [YS3]
  Demux/2 -> [YS2]
  Demux/4 -> [YS4]
  Demux/5 -> [YS5]
  Demux/6 -> [YS6]
  Demux/7 -> [YS10]
  Demux/8 -> [YS20]
  Demux/9 -> [YS30]
  Demux/10 -> [YS40]
  Demux/11 -> [YS50]
  Demux/12 -> [YS60]

== system motorl/STAR/PULSE/B1/LOOKUP TABLE/If Action Subsystem ==
  In1 : Inport
  Action Port : ActionPort  ActionType=case
  Out1 : Outport
  wires:
  In1/1 -> Out1/1

== system motorl/STAR/PULSE/B1/LOOKUP TABLE/If Action Subsystem1 ==
  In1 : Inport
  Action Port : ActionPort  ActionType=case
  Out1 : Outport
  wires:
  In1/1 -> Out1/1

== system motorl/STAR/PULSE/B1/LOOKUP TABLE/If Action Subsystem10 ==
  In1 : Inport
  Action Port : ActionPort  ActionType=case
  Out1 : Outport
  wires:
  In1/1 -> Out1/1

== system motorl/STAR/PULSE/B1/LOOKUP TABLE/If Action Subsystem2 ==
  In1 : Inport
  Action Port : ActionPort  ActionType=case
  Out1 : Outport
  wires:
  In1/1 -> Out1/1

== system motorl/STAR/PULSE/B1/LOOKUP TABLE/If Action Subsystem3 ==
  In1 : Inport
  Action Port : ActionPort  ActionType=case
  Out1 : Outport
  wires:
  In1/1 -> Out1/1

== system motorl/STAR/PULSE/B1/LOOKUP TABLE/If Action Subsystem4 ==
  In1 : Inport
  Action Port : ActionPort  ActionType=case
  Out1 : Outport
  wires:
  In1/1 -> Out1/1

== system motorl/STAR/PULSE/B1/LOOKUP TABLE/If Action Subsystem5 ==
  In1 : Inport
  Action Port : ActionPort  ActionType=case
  Out1 : Outport
  wires:
  In1/1 -> Out1/1

== system motorl/STAR/PULSE/B1/LOOKUP TABLE/If Action Subsystem6 ==
  In1 : Inport
  Action Port : ActionPort  ActionType=case
  Out1 : Outport
  wires:
  In1/1 -> Out1/1

== system motorl/STAR/PULSE/B1/LOOKUP TABLE/If Action Subsystem7 ==
  In1 : Inport
  Action Port : ActionPort  ActionType=case
  Out1 : Outport
  wires:
  In1/1 -> Out1/1

== system motorl/STAR/PULSE/B1/LOOKUP TABLE/If Action Subsystem8 ==
  In1 : Inport
  Action Port : ActionPort  ActionType=case
  Out1 : Outport
  wires:
  In1/1 -> Out1/1

== system motorl/STAR/PULSE/B1/LOOKUP TABLE/If Action Subsystem9 ==
  In1 : Inport
  Action Port : ActionPort  ActionType=case
  Out1 : Outport
  wires:
  In1/1 -> Out1/1

== system motorl/STAR/PULSE/R1/LOOKUP TABLE/If Action Subsystem ==
  In1 : Inport
  Action Port : ActionPort  ActionType=case
  Out1 : Outport
  wires:
  In1/1 -> Out1/1

== system motorl/STAR/PULSE/R1/LOOKUP TABLE/If Action Subsystem1 ==
  In1 : Inport
  Action Port : ActionPort  ActionType=case
  Out1 : Outport
  wires:
  In1/1 -> Out1/1

== system motorl/STAR/PULSE/R1/LOOKUP TABLE/If Action Subsystem10 ==
  In1 : Inport
  Action Port : ActionPort  ActionType=case
  Out1 : Outport
  wires:
  In1/1 -> Out1/1

== system motorl/STAR/PULSE/R1/LOOKUP TABLE/If Action Subsystem2 ==
  In1 : Inport
  Action Port : ActionPort  ActionType=case
  Out1 : Outport
  wires:
  In1/1 -> Out1/1

== system motorl/STAR/PULSE/R1/LOOKUP TABLE/If Action Subsystem3 ==
  In1 : Inport
  Action Port : ActionPort  ActionType=case
  Out1 : Outport
  wires:
  In1/1 -> Out1/1

== system motorl/STAR/PULSE/R1/LOOKUP TABLE/If Action Subsystem4 ==
  In1 : Inport
  Action Port : ActionPort  ActionType=case
  Out1 : Outport
  wires:
  In1/1 -> Out1/1

== system motorl/STAR/PULSE/R1/LOOKUP TABLE/If Action Subsystem5 ==
  In1 : Inport
  Action Port : ActionPort  ActionType=case
  Out1 : Outport
  wires:
  In1/1 -> Out1/1

== system motorl/STAR/PULSE/R1/LOOKUP TABLE/If Action Subsystem6 ==
  In1 : Inport
  Action Port : ActionPort  ActionType=case
  Out1 : Outport
  wires:
  In1/1 -> Out1/1

== system motorl/STAR/PULSE/R1/LOOKUP TABLE/If Action Subsystem7 ==
  In1 : Inport
  Action Port : ActionPort  ActionType=case
  Out1 : Outport
  wires:
  In1/1 -> Out1/1

== system motorl/STAR/PULSE/R1/LOOKUP TABLE/If Action Subsystem8 ==
  In1 : Inport
  Action Port : ActionPort  ActionType=case
  Out1 : Outport
  wires:
  In1/1 -> Out1/1

== system motorl/STAR/PULSE/R1/LOOKUP TABLE/If Action Subsystem9 ==
  In1 : Inport
  Action Port : ActionPort  ActionType=case
  Out1 : Outport
  wires:
  In1/1 -> Out1/1

== system motorl/STAR/PULSE/Y1/LOOKUP TABLE/If Action Subsystem ==
  In1 : Inport
  Action Port : ActionPort  ActionType=case
  Out1 : Outport
  wires:
  In1/1 -> Out1/1

== system motorl/STAR/PULSE/Y1/LOOKUP TABLE/If Action Subsystem1 ==
  In1 : Inport
  Action Port : ActionPort  ActionType=case
  Out1 : Outport
  wires:
  In1/1 -> Out1/1

== system motorl/STAR/PULSE/Y1/LOOKUP TABLE/If Action Subsystem10 ==
  In1 : Inport
  Action Port : ActionPort  ActionType=case
  Out1 : Outport
  wires:
  In1/1 -> Out1/1

== system motorl/STAR/PULSE/Y1/LOOKUP TABLE/If Action Subsystem2 ==
  In1 : Inport
  Action Port : ActionPort  ActionType=case
  Out1 : Outport
  wires:
  In1/1 -> Out1/1

== system motorl/STAR/PULSE/Y1/LOOKUP TABLE/If Action Subsystem3 ==
  In1 : Inport
  Action Port : ActionPort  ActionType=case
  Out1 : Outport
  wires:
  In1/1 -> Out1/1

== system motorl/STAR/PULSE/Y1/LOOKUP TABLE/If Action Subsystem4 ==
  In1 : Inport
  Action Port : ActionPort  ActionType=case
  Out1 : Outport
  wires:
  In1/1 -> Out1/1

== system motorl/STAR/PULSE/Y1/LOOKUP TABLE/If Action Subsystem5 ==
  In1 : Inport
  Action Port : ActionPort  ActionType=case
  Out1 : Outport
  wires:
  In1/1 -> Out1/1

== system motorl/STAR/PULSE/Y1/LOOKUP TABLE/If Action Subsystem6 ==
  In1 : Inport
  Action Port : ActionPort  ActionType=case
  Out1 : Outport
  wires:
  In1/1 -> Out1/1

== system motorl/STAR/PULSE/Y1/LOOKUP TABLE/If Action Subsystem7 ==
  In1 : Inport
  Action Port : ActionPort  ActionType=case
  Out1 : Outport
  wires:
  In1/1 -> Out1/1

== system motorl/STAR/PULSE/Y1/LOOKUP TABLE/If Action Subsystem8 ==
  In1 : Inport
  Action Port : ActionPort  ActionType=case
  Out1 : Outport
  wires:
  In1/1 -> Out1/1

== system motorl/STAR/PULSE/Y1/LOOKUP TABLE/If Action Subsystem9 ==
  In1 : Inport
  Action Port : ActionPort  ActionType=case
  Out1 : Outport
  wires:
  In1/1 -> Out1/1
